simulink model "TorqueAllocatorTestWrapper"  (R2026b)
settings: Solver=FixedStepDiscrete  StopTime=0.1  FixedStep=UnifiedControlSampleTime
settings Model: DataDictionary=VehicleData.sldd  Creator=Xu Dingyi  LastModifiedBy=29358

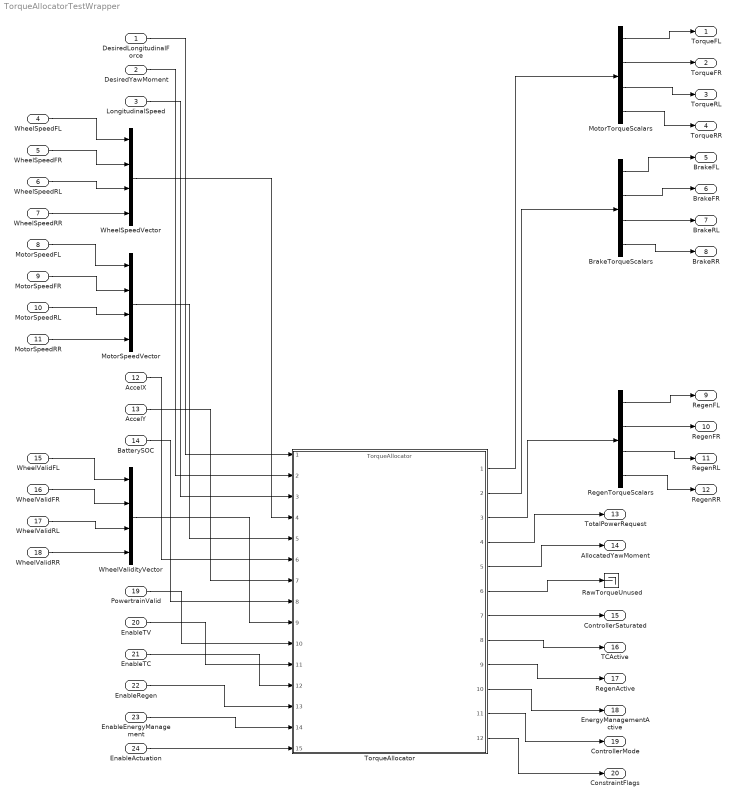
== system TorqueAllocatorTestWrapper ==
  DesiredLongitudinalForce : Inport  OutDataTypeStr=double
  DesiredYawMoment : Inport  Port=2  OutDataTypeStr=double
  LongitudinalSpeed : Inport  Port=3  OutDataTypeStr=double
  WheelSpeedFL : Inport  Port=4  OutDataTypeStr=double
  WheelSpeedFR : Inport  Port=5  OutDataTypeStr=double
  WheelSpeedRL : Inport  Port=6  OutDataTypeStr=double
  WheelSpeedRR : Inport  Port=7  OutDataTypeStr=double
  MotorSpeedFL : Inport  Port=8  OutDataTypeStr=double
  MotorSpeedFR : Inport  Port=9  OutDataTypeStr=double
  MotorSpeedRL : Inport  Port=10  OutDataTypeStr=double
  MotorSpeedRR : Inport  Port=11  OutDataTypeStr=double
  AccelX : Inport  Port=12  OutDataTypeStr=double
  AccelY : Inport  Port=13  OutDataTypeStr=double
  BatterySOC : Inport  Port=14  OutDataTypeStr=double
  WheelValidFL : Inport  Port=15  OutDataTypeStr=boolean
  WheelValidFR : Inport  Port=16  OutDataTypeStr=boolean
  WheelValidRL : Inport  Port=17  OutDataTypeStr=boolean
  WheelValidRR : Inport  Port=18  OutDataTypeStr=boolean
  PowertrainValid : Inport  Port=19  OutDataTypeStr=boolean
  EnableTV : Inport  Port=20  OutDataTypeStr=boolean
  EnableTC : Inport  Port=21  OutDataTypeStr=boolean
  EnableRegen : Inport  Port=22  OutDataTypeStr=boolean
  EnableEnergyManagement : Inport  Port=23  OutDataTypeStr=boolean
  EnableActuation : Inport  Port=24  OutDataTypeStr=boolean
  BrakeTorqueScalars : Demux
  MotorSpeedVector : Mux
  MotorTorqueScalars : Demux
  RawTorqueUnused : Terminator
  RegenTorqueScalars : Demux
  TorqueAllocator : ModelReference  ModelNameDialog=TorqueAllocator  ModelReferenceVersion=2.0
  WheelSpeedVector : Mux
  WheelValidityVector : Mux
  TorqueFL : Outport  OutDataTypeStr=double
  TorqueFR : Outport  Port=2  OutDataTypeStr=double
  TorqueRL : Outport  Port=3  OutDataTypeStr=double
  TorqueRR : Outport  Port=4  OutDataTypeStr=double
  BrakeFL : Outport  Port=5  OutDataTypeStr=double
  BrakeFR : Outport  Port=6  OutDataTypeStr=double
  BrakeRL : Outport  Port=7  OutDataTypeStr=double
  BrakeRR : Outport  Port=8  OutDataTypeStr=double
  RegenFL : Outport  Port=9  OutDataTypeStr=double
  RegenFR : Outport  Port=10  OutDataTypeStr=double
  RegenRL : Outport  Port=11  OutDataTypeStr=double
  RegenRR : Outport  Port=12  OutDataTypeStr=double
  TotalPowerRequest : Outport  Port=13  OutDataTypeStr=double
  AllocatedYawMoment : Outport  Port=14  OutDataTypeStr=double
  ControllerSaturated : Outport  Port=15  OutDataTypeStr=boolean
  TCActive : Outport  Port=16  OutDataTypeStr=boolean
  RegenActive : Outport  Port=17  OutDataTypeStr=boolean
  EnergyManagementActive : Outport  Port=18  OutDataTypeStr=boolean
  ControllerMode : Outport  Port=19  OutDataTypeStr=uint8
  ConstraintFlags : Outport  Port=20  OutDataTypeStr=uint16
  wires:
  WheelSpeedFL/1 -> WheelSpeedVector/1
  TorqueAllocator/8 -> TCActive/1
  TorqueAllocator/7 -> ControllerSaturated/1
  MotorSpeedFL/1 -> MotorSpeedVector/1
  AccelX/1 -> TorqueAllocator/6
  WheelSpeedFR/1 -> WheelSpeedVector/2
  TorqueAllocator/4 -> TotalPowerRequest/1
  TorqueAllocator/1 -> MotorTorqueScalars/1
  WheelSpeedRL/1 -> WheelSpeedVector/3
  LongitudinalSpeed/1 -> TorqueAllocator/3
  MotorSpeedRR/1 -> MotorSpeedVector/4
  RegenTorqueScalars/2 -> RegenFR/1
  WheelSpeedRR/1 -> WheelSpeedVector/4
  MotorSpeedFR/1 -> MotorSpeedVector/2
  DesiredYawMoment/1 -> TorqueAllocator/2
  MotorSpeedRL/1 -> MotorSpeedVector/3
  BatterySOC/1 -> TorqueAllocator/8
  WheelSpeedVector/1 -> TorqueAllocator/4
  WheelValidFL/1 -> WheelValidityVector/1
  WheelValidFR/1 -> WheelValidityVector/2
  BrakeTorqueScalars/3 -> BrakeRL/1
  BrakeTorqueScalars/2 -> BrakeFR/1
  WheelValidRL/1 -> WheelValidityVector/3
  TorqueAllocator/10 -> EnergyManagementActive/1
  TorqueAllocator/9 -> RegenActive/1
  PowertrainValid/1 -> TorqueAllocator/10
  WheelValidRR/1 -> WheelValidityVector/4
  TorqueAllocator/6 -> RawTorqueUnused/1
  TorqueAllocator/5 -> AllocatedYawMoment/1
  DesiredLongitudinalForce/1 -> TorqueAllocator/1
  MotorSpeedVector/1 -> TorqueAllocator/5
  AccelY/1 -> TorqueAllocator/7
  WheelValidityVector/1 -> TorqueAllocator/9
  EnableTV/1 -> TorqueAllocator/11
  MotorTorqueScalars/2 -> TorqueFR/1
  MotorTorqueScalars/1 -> TorqueFL/1
  EnableTC/1 -> TorqueAllocator/12
  EnableRegen/1 -> TorqueAllocator/13
  TorqueAllocator/11 -> ControllerMode/1
  EnableEnergyManagement/1 -> TorqueAllocator/14
  EnableActuation/1 -> TorqueAllocator/15
  TorqueAllocator/3 -> RegenTorqueScalars/1
  TorqueAllocator/2 -> BrakeTorqueScalars/1
  TorqueAllocator/12 -> ConstraintFlags/1
  MotorTorqueScalars/4 -> TorqueRR/1
  MotorTorqueScalars/3 -> TorqueRL/1
  BrakeTorqueScalars/4 -> BrakeRR/1
  BrakeTorqueScalars/1 -> BrakeFL/1
  RegenTorqueScalars/1 -> RegenFL/1
  RegenTorqueScalars/3 -> RegenRL/1
  RegenTorqueScalars/4 -> RegenRR/1
